simulink subsystem "consensusPump"  (R2022b)
settings: Solver=VariableStepAuto  StartTime=0.0  StopTime=10.0  RelTol=1e-3
model mask{n_unit=0}
  mask prompts: n_unit "n_unit value"
undefined symbols (not defined in the file): c
settings Model: Creator=is123  LastModifiedBy=is123

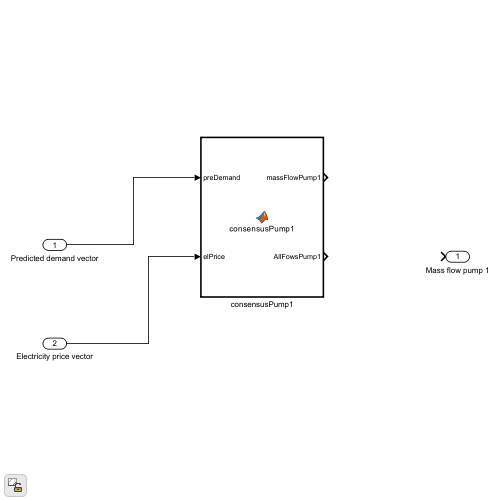
[thumbnail: Simulink's stored preview of the top-level diagram]
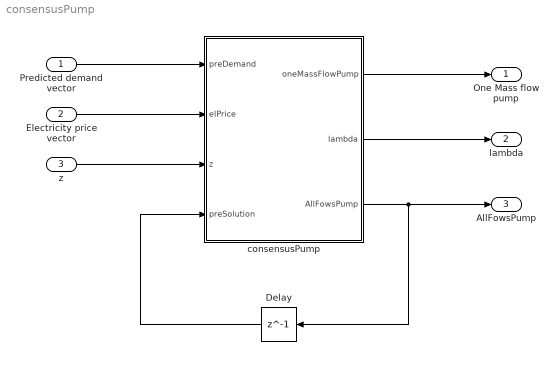
== system consensusPump ==
  Predicted demand vector : Inport
  Electricity price vector : Inport  Port=2
  z : Inport  Port=3
  Delay : Delay  DelayLength=1  InitialCondition=zeros(c.Nu*c.Nc,1)
  consensusPump : MATLAB Function  TreatAsAtomicUnit=on  SystemSampleTime=3600/c.AccTime
  "One Mass flow pump " : Outport
  lambda : Outport  Port=2
  "AllFowsPump " : Outport  Port=3
  wires:
  Predicted demand vector/1 -> consensusPump/1(preDemand)
  Electricity price vector/1 -> consensusPump/2(elPrice)
  consensusPump/1(oneMassFlowPump) -> "One Mass flow pump "/1
  consensusPump/3(AllFowsPump) -> Delay/1, "AllFowsPump "/1
  z/1 -> consensusPump/3(z)
  Delay/1 -> consensusPump/4(preSolution)
  consensusPump/2(lambda) -> lambda/1

== matlab function consensusPump/consensusPump ==
  data: preDemand input; oneMassFlowPump output; lambda output; AllFowsPump output; elPrice input; z input; preSolution input
function [oneMassFlowPump,lambda,AllFowsPump] = consensusPump(preDemand, elPrice,z,preSolution)

y = u;
